simulink model "y_heli"  (R2016b)
settings: Solver=VariableStepAuto  StartTime=0.0  StopTime=50  RelTol=1e-3
values from neighbouring files (symbols this model uses):
  SAT_INT_ERR_PITCH = 5    [setup_lab_heli_2d.m]
  SAT_INT_ERR_YAW = 5    [setup_lab_heli_2d.m]
  Tr_p = 1    [setup_lab_heli_2d.m]
  Tr_y = 1    [setup_lab_heli_2d.m]
undefined symbols (not defined in the file or in its folder): Ki
libraries: simulink_extras x4, heli_2d_lib x2
settings Model: Creator=luy0a  LastModifiedBy=luy0a

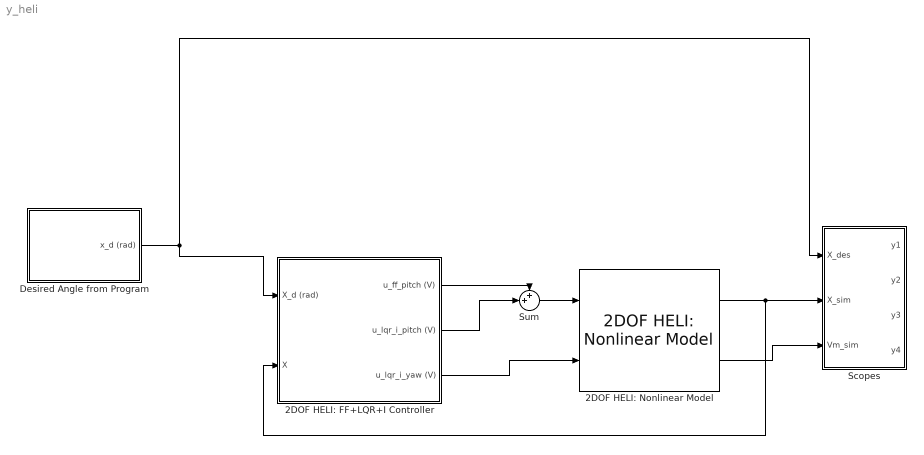
== system y_heli ==
  2DOF HELI: FF+LQR+I Controller : Subsystem  AncestorBlock=heli_2d_lib/2DOF HELI: FF+LQR+I Controller
  2DOF HELI: Nonlinear Model : heli_2d_lib/2DOF HELI: Nonlinear Model
  Desired Angle from Program : Subsystem
  Scopes : Subsystem  AncestorBlock=heli_2d_lib/Scopes
  Sum : Sum  Inputs=++|
  wires:
  Desired Angle from Program/1(x_d (rad)) -> 2DOF HELI: FF+LQR+I Controller/1(X_d (rad)), Scopes/1(X_des)
  2DOF HELI: Nonlinear Model/1 -> 2DOF HELI: FF+LQR+I Controller/2(X), Scopes/2(X_sim)
  2DOF HELI: Nonlinear Model/2 -> Scopes/3(Vm_sim)
  2DOF HELI: FF+LQR+I Controller/1(u_ff_pitch (V)) -> Sum/1
  Sum/1 -> 2DOF HELI: Nonlinear Model/1
  2DOF HELI: FF+LQR+I Controller/2(u_lqr_i_pitch (V)) -> Sum/2
  2DOF HELI: FF+LQR+I Controller/3(u_lqr_i_yaw (V)) -> 2DOF HELI: Nonlinear Model/2

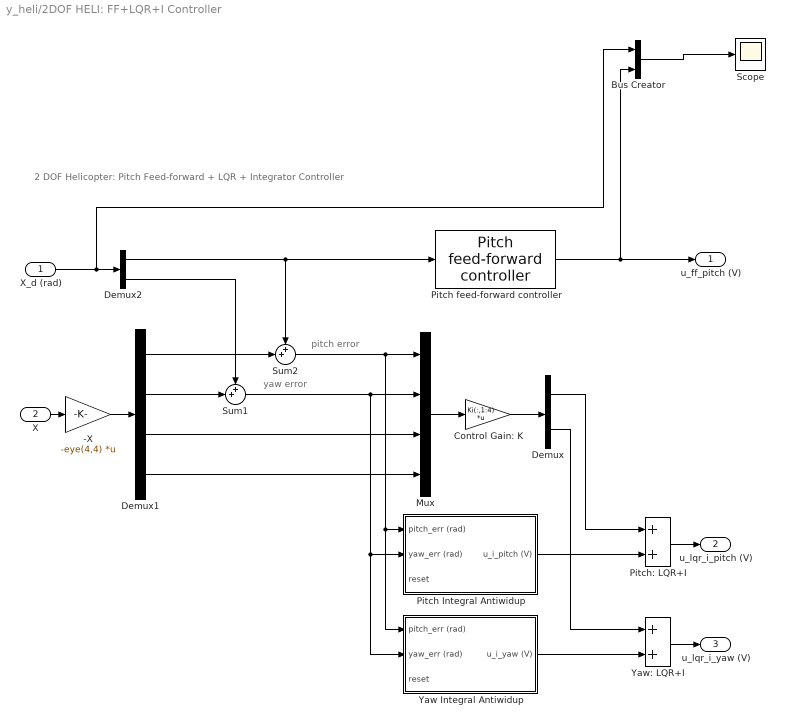
== system y_heli/2DOF HELI: FF+LQR+I Controller ==
  note: yaw error
  note: pitch error
  note: 2 DOF Helicopter:
      | Pitch Feed-forward + LQR + Integrator Controller
  X_d (rad) : Inport
  X : Inport  Port=2
  -X : Gain  Gain=-eye(4,4)  Multiplication=Matrix(K*u)
  Bus Creator : BusCreator  Inputs=2
  Control Gain: K : Gain  Gain=Ki(:,1:4)  Multiplication=Matrix(K*u)
  Demux : Demux  Outputs=2
  Demux1 : Demux
  Demux2 : Demux  Outputs=2
  Mux : Mux
  Pitch Integral Antiwidup : Subsystem  AncestorBlock=heli_2d_lib/2DOF HELI: FF+LQR+I Controller/Yaw Integral Antiwidup
  Pitch feed-forward controller : heli_2d_lib/Pitch feed-forward controller
  Pitch: LQR+I : Sum
  Scope : Scope
  Sum1 : Sum  Inputs=++|
  Sum2 : Sum  Inputs=++|
  Yaw Integral Antiwidup : Subsystem
  Yaw: LQR+I : Sum
  u_ff_pitch (V) : Outport
  u_lqr_i_pitch (V) : Outport  Port=2
  u_lqr_i_yaw (V) : Outport  Port=3
  wires:
  Bus Creator/1 -> Scope/1
  Demux1/2 -> Sum1/2
  Demux2/2 -> Sum1/1
  Demux2/1 -> Sum2/1, Pitch feed-forward controller/1
  X_d (rad)/1 -> Demux2/1, Bus Creator/1
  Yaw Integral Antiwidup/1(u_i_yaw (V)) -> Yaw: LQR+I/2
  Demux/2 -> Yaw: LQR+I/1
  Yaw: LQR+I/1 -> u_lqr_i_yaw (V)/1
  Pitch: LQR+I/1 -> u_lqr_i_pitch (V)/1
  Demux/1 -> Pitch: LQR+I/1
  Pitch Integral Antiwidup/1(u_i_pitch (V)) -> Pitch: LQR+I/2
  Pitch feed-forward controller/1 -> Bus Creator/2, u_ff_pitch (V)/1
  Sum2/1 -> Mux/1, Yaw Integral Antiwidup/1(pitch_err (rad)), Pitch Integral Antiwidup/1(pitch_err (rad))
  Demux1/1 -> Sum2/2
  X/1 -> -X/1
  Sum1/1 -> Yaw Integral Antiwidup/2(yaw_err (rad)), Pitch Integral Antiwidup/2(yaw_err (rad)), Mux/2
  -X/1 -> Demux1/1
  Control Gain: K/1 -> Demux/1
  Mux/1 -> Control Gain: K/1
  Demux1/3 -> Mux/3
  Demux1/4 -> Mux/4

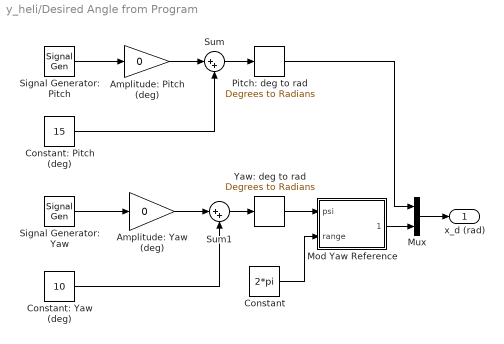
== system y_heli/Desired Angle from Program ==
  Amplitude: Pitch (deg) : Gain  Gain=0
  Amplitude: Yaw (deg) : Gain  Gain=0
  Constant : Constant  Value=2*pi
  Constant: Pitch (deg) : Constant  Value=15
  Constant: Yaw (deg) : Constant  Value=10
  Mod Yaw Reference : Subsystem
  Mux : Mux  Inputs=2
  Pitch: deg to rad : simulink_extras/Transformations/Degrees to Radians
  Signal Generator: Pitch : SignalGenerator  WaveForm=square  Frequency=0.05
  Signal Generator: Yaw : SignalGenerator  WaveForm=square  Frequency=0.05
  Sum : Sum  Inputs=|++
  Sum1 : Sum  Inputs=|++
  Yaw: deg to rad : simulink_extras/Transformations/Degrees to Radians
  x_d (rad) : Outport
  wires:
  Mux/1 -> x_d (rad)/1
  Constant: Yaw (deg)/1 -> Sum1/2
  Amplitude: Yaw (deg)/1 -> Sum1/1
  Signal Generator: Yaw/1 -> Amplitude: Yaw (deg)/1
  Sum1/1 -> Yaw: deg to rad/1
  Constant: Pitch (deg)/1 -> Sum/2
  Amplitude: Pitch (deg)/1 -> Sum/1
  Signal Generator: Pitch/1 -> Amplitude: Pitch (deg)/1
  Sum/1 -> Pitch: deg to rad/1
  Pitch: deg to rad/1 -> Mux/1
  Mod Yaw Reference/1(mod psi) -> Mux/2
  Yaw: deg to rad/1 -> Mod Yaw Reference/1(psi)
  Constant/1 -> Mod Yaw Reference/2(range)

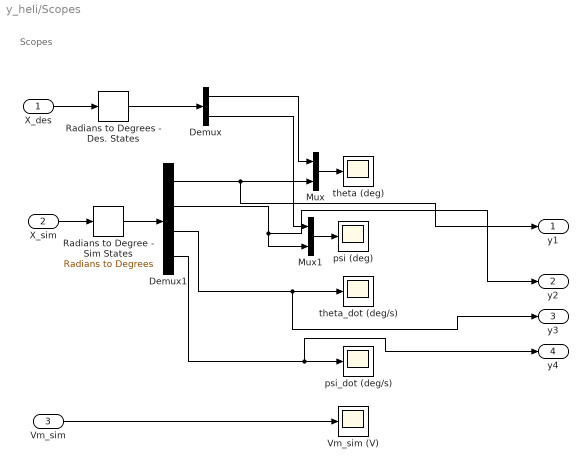
== system y_heli/Scopes ==
  note: Scopes
  X_des : Inport
  X_sim : Inport  Port=2
  Vm_sim : Inport  Port=3
  Demux : Demux  Outputs=2
  Demux1 : Demux
  Mux : Mux  Inputs=2
  Mux1 : Mux  Inputs=2
  Radians to Degree - Sim States : simulink_extras/Transformations/Radians to Degrees
  Radians to Degrees - Des. States : simulink_extras/Transformations/Radians to Degrees
  Vm_sim (V) : Scope
  psi (deg) : Scope
  psi_dot (deg/s) : Scope
  theta (deg) : Scope
  theta_dot (deg/s) : Scope
  y1 : Outport
  y2 : Outport  Port=2
  y3 : Outport  Port=3
  y4 : Outport  Port=4
  wires:
  Demux1/4 -> y4/1, psi_dot (deg/s)/1
  Demux1/3 -> y3/1, theta_dot (deg/s)/1
  Mux1/1 -> psi (deg)/1
  Mux/1 -> theta (deg)/1
  Radians to Degree - Sim States/1 -> Demux1/1
  X_sim/1 -> Radians to Degree - Sim States/1
  X_des/1 -> Radians to Degrees - Des. States/1
  Demux/1 -> Mux/1
  Demux1/1 -> y1/1, Mux/2
  Demux/2 -> Mux1/1
  Demux1/2 -> y2/1, Mux1/2
  Radians to Degrees - Des. States/1 -> Demux/1
  Vm_sim/1 -> Vm_sim (V)/1

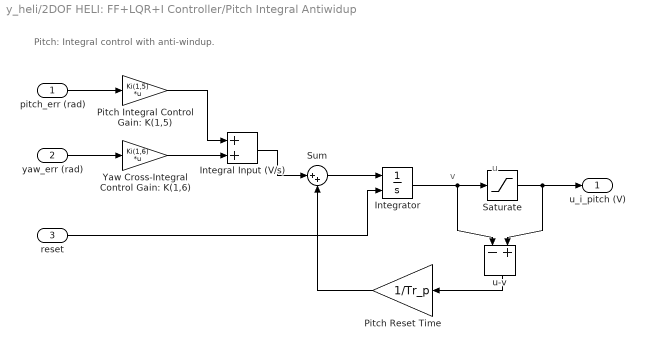
== system y_heli/2DOF HELI: FF+LQR+I Controller/Pitch Integral Antiwidup ==
  note: Pitch: Integral control with anti-windup.
  note: v
  note: u
  pitch_err (rad) : Inport
  yaw_err (rad) : Inport  Port=2
  reset : Inport  Port=3
  Integral Input (V/s) : Sum
  Integrator : Integrator  ExternalReset=rising
  Pitch Integral Control Gain: K(1,5) : Gain  Gain=Ki(1,5)  Multiplication=Matrix(K*u)
  Pitch Reset Time : Gain  Gain=1/Tr_p
  Saturate : Saturate  UpperLimit=SAT_INT_ERR_PITCH  LowerLimit=-SAT_INT_ERR_PITCH
  Sum : Sum  Inputs=|++
  Yaw Cross-Integral Control Gain: K(1,6) : Gain  Gain=Ki(1,6)  Multiplication=Matrix(K*u)
  u-v : Sum  Inputs=-+
  u_i_pitch (V) : Outport
  wires:
  Integral Input (V/s)/1 -> Sum/1
  Yaw Cross-Integral Control Gain: K(1,6)/1 -> Integral Input (V/s)/2
  Pitch Integral Control Gain: K(1,5)/1 -> Integral Input (V/s)/1
  yaw_err (rad)/1 -> Yaw Cross-Integral Control Gain: K(1,6)/1
  reset/1 -> Integrator/2
  Pitch Reset Time/1 -> Sum/2
  Sum/1 -> Integrator/1
  u-v/1 -> Pitch Reset Time/1
  Saturate/1 -> u-v/2, u_i_pitch (V)/1
  Integrator/1 -> Saturate/1, u-v/1
  pitch_err (rad)/1 -> Pitch Integral Control Gain: K(1,5)/1

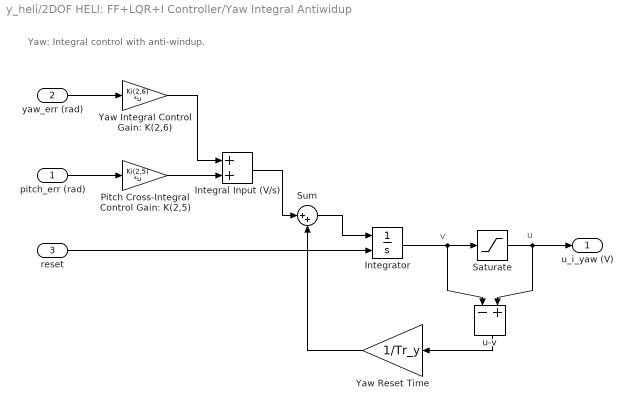
== system y_heli/2DOF HELI: FF+LQR+I Controller/Yaw Integral Antiwidup ==
  note: Yaw: Integral control with anti-windup.
  note: u
  note: v
  pitch_err (rad) : Inport
  yaw_err (rad) : Inport  Port=2
  reset : Inport  Port=3
  Integral Input (V/s) : Sum
  Integrator : Integrator  ExternalReset=rising
  Pitch Cross-Integral Control Gain: K(2,5) : Gain  Gain=Ki(2,5)  Multiplication=Matrix(K*u)
  Saturate : Saturate  UpperLimit=SAT_INT_ERR_YAW  LowerLimit=-SAT_INT_ERR_YAW
  Sum : Sum  Inputs=|++
  Yaw Integral Control Gain: K(2,6) : Gain  Gain=Ki(2,6)  Multiplication=Matrix(K*u)
  Yaw Reset Time : Gain  Gain=1/Tr_y
  u-v : Sum  Inputs=-+
  u_i_yaw (V) : Outport
  wires:
  Integral Input (V/s)/1 -> Sum/1
  Pitch Cross-Integral Control Gain: K(2,5)/1 -> Integral Input (V/s)/2
  Yaw Integral Control Gain: K(2,6)/1 -> Integral Input (V/s)/1
  pitch_err (rad)/1 -> Pitch Cross-Integral Control Gain: K(2,5)/1
  reset/1 -> Integrator/2
  yaw_err (rad)/1 -> Yaw Integral Control Gain: K(2,6)/1
  Integrator/1 -> u-v/1, Saturate/1
  Saturate/1 -> u_i_yaw (V)/1, u-v/2
  u-v/1 -> Yaw Reset Time/1
  Sum/1 -> Integrator/1
  Yaw Reset Time/1 -> Sum/2

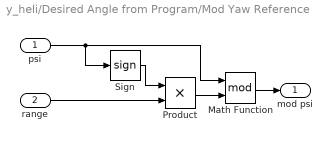
== system y_heli/Desired Angle from Program/Mod Yaw Reference ==
  psi : Inport
  range : Inport  Port=2
  Math Function : Math  Operator=mod  SaturateOnIntegerOverflow=on
  Product : Product  RndMeth=Zero
  Sign : Signum
  mod psi : Outport
  wires:
  Product/1 -> Math Function/2
  Sign/1 -> Product/1
  psi/1 -> Math Function/1, Sign/1
  Math Function/1 -> mod psi/1
  range/1 -> Product/2
